simulink model "UAM_GuidanceAndNavigation"  (R2024b)
settings: Solver=VariableStepAuto  StartTime=0.0  StopTime=10.0  RelTol=1e-3
undefined symbols (not defined in the file): Earth, WGS84
libraries: robotcorelib x2, simulink x1, uavalgslib x1, mspfiltlib x1, simulink_extras x1, aerolibtransform2 x1
settings Model: DataDictionary=UAM_data.sldd  Creator=admin  LastModifiedBy=USER

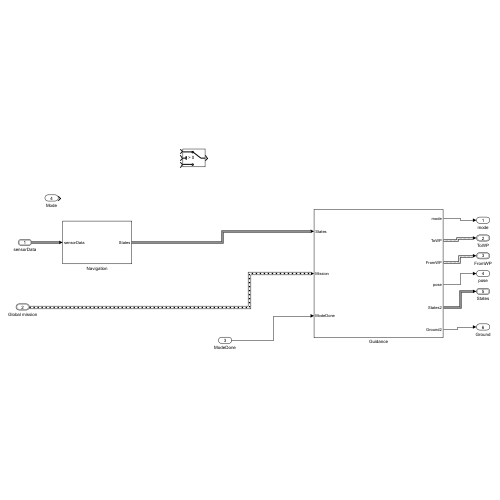
[thumbnail: Simulink's stored preview of the top-level diagram]
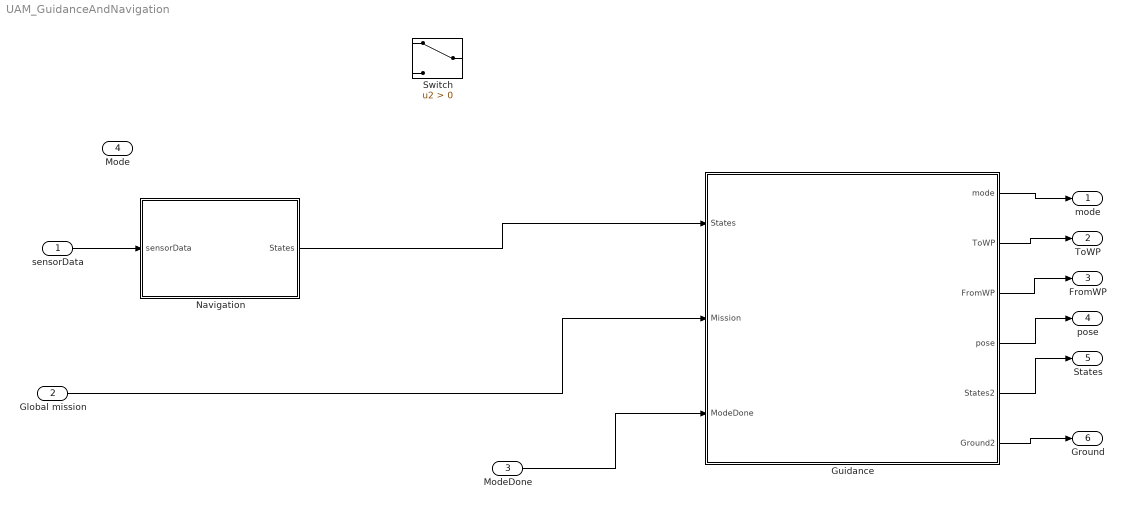
== system UAM_GuidanceAndNavigation ==
  sensorData : Inport  OutDataTypeStr=Bus: sensorData
  Global mission : Inport  Port=2  OutDataTypeStr=Bus: UAVPathManagerBus  PortDimensions=9  BusOutputAsStruct=on
  ModeDone : Inport  Port=3  OutDataTypeStr=uint8
  Mode : Inport  Port=4  OutDataTypeStr=Enum: FlightModeType
  Guidance : Subsystem
  Navigation : Subsystem
  Switch : Switch  Criteria=u2 > Threshold  SaturateOnIntegerOverflow=off  InputSameDT=off
  mode : Outport  BusOutputAsStruct=on
  ToWP : Outport  Port=2  OutDataTypeStr=Bus: UAVPathManagerBus
  FromWP : Outport  Port=3  OutDataTypeStr=Bus: UAVPathManagerBus
  pose : Outport  Port=4
  States : Outport  Port=5  OutDataTypeStr=Bus: GuidanceStates
  Ground : Outport  Port=6
  wires:
  Global mission/1 -> Guidance/2(Mission)
  Navigation/1(States) -> Guidance/1(States)
  sensorData/1 -> Navigation/1(sensorData)
  Guidance/1(mode) -> mode/1
  Guidance/2(ToWP) -> ToWP/1
  Guidance/3(FromWP) -> FromWP/1
  Guidance/4(pose) -> pose/1
  Guidance/5(States2) -> States/1
  Guidance/6(Ground2) -> Ground/1
  ModeDone/1 -> Guidance/3(ModeDone)

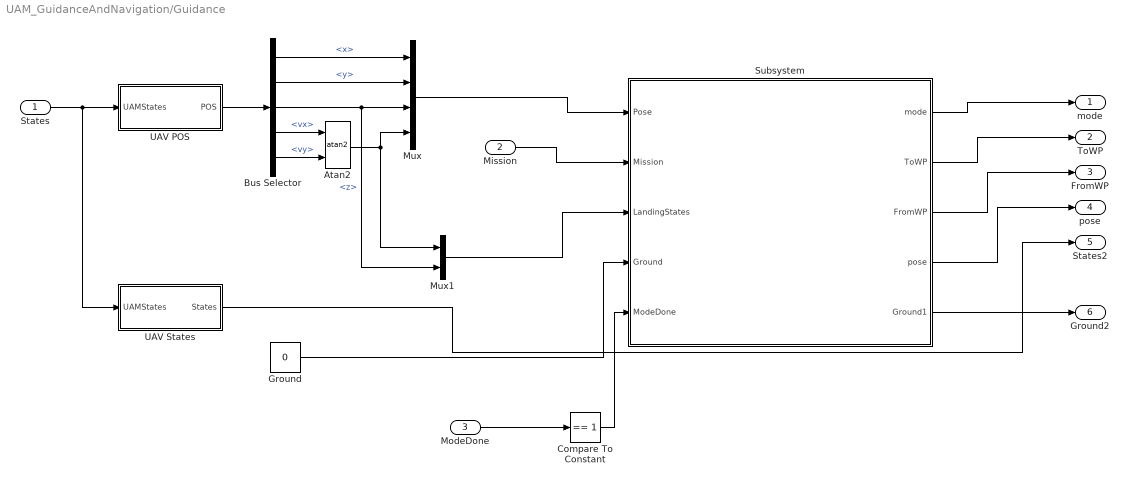
== system UAM_GuidanceAndNavigation/Guidance ==
  States : Inport  OutDataTypeStr=Bus: StateBus
  Mission : Inport  Port=2  OutDataTypeStr=Bus: UAVPathManagerBus
  ModeDone : Inport  Port=3
  Atan2 : Trigonometry  Operator=atan2
  Bus Selector : BusSelector  OutputSignals=x,y,z,vx,vy
  Compare To Constant : simulink/Logic and Bit Operations/Compare To Constant  relop===  const=1  OutDataTypeStr=boolean
  Ground : Constant  Value=0
  Mux : Mux
  Mux1 : Mux  Inputs=2
  Subsystem : Subsystem
  UAV POS : Subsystem
  UAV States : Subsystem
  mode : Outport
  ToWP : Outport  Port=2
  FromWP : Outport  Port=3
  pose : Outport  Port=4
  States2 : Outport  Port=5  OutDataTypeStr=Bus: GuidanceStates
  Ground2 : Outport  Port=6
  wires:
  UAV POS/1(POS) -> Bus Selector/1
  States/1 -> UAV States/1(UAMStates), UAV POS/1(UAMStates)
  Bus Selector/5 -> Atan2/2  "<vy>"
  Bus Selector/4 -> Atan2/1  "<vx>"
  Bus Selector/1 -> Mux/1  "<x>"
  Bus Selector/2 -> Mux/2  "<y>"
  Bus Selector/3 -> Mux1/2, Mux/3  "<z>"
  Atan2/1 -> Mux1/1, Mux/4
  Ground/1 -> Subsystem/4(Ground)
  Mux/1 -> Subsystem/1(Pose)
  Mux1/1 -> Subsystem/3(LandingStates)
  Mission/1 -> Subsystem/2(Mission)
  Subsystem/1(mode) -> mode/1
  Subsystem/5(Ground1) -> Ground2/1
  UAV States/1(States) -> States2/1
  Subsystem/4(pose) -> pose/1
  Subsystem/3(FromWP) -> FromWP/1
  Subsystem/2(ToWP) -> ToWP/1
  ModeDone/1 -> Compare To Constant/1
  Compare To Constant/1 -> Subsystem/5(ModeDone)

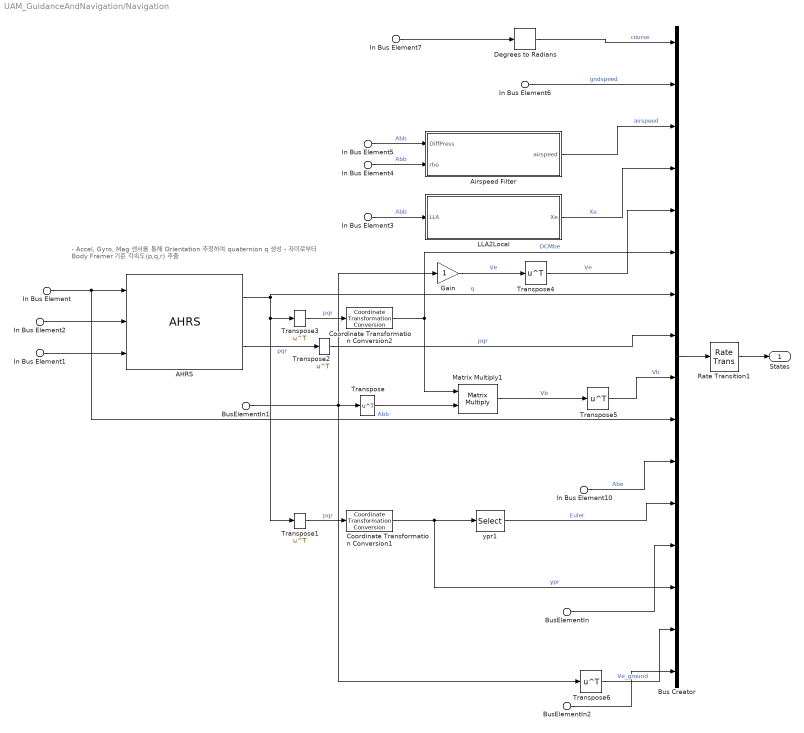
== system UAM_GuidanceAndNavigation/Navigation ==
  note: - Accel, Gyro, Mag 센서를 통해 Orientation 추정하여 quaternion q 생성
      | - 자이로부터 Body Framer 기준 각속도(p,q,r) 추출
  In Bus Element3 : Inport  PortName=sensorData  Element=LLA
  In Bus Element : Inport  PortName=sensorData  Element=Abb
  In Bus Element2 : Inport  PortName=sensorData  Element=Gyro
  In Bus Element1 : Inport  PortName=sensorData  Element=Mag
  BusElementIn1 : Inport  PortName=sensorData  Element=GPSVelocity
  In Bus Element10 : Inport  PortName=sensorData  Element=Abe
  BusElementIn : Inport  PortName=sensorData  Element=RotorParameter
  In Bus Element7 : Inport  PortName=sensorData  Element=GPSCourse
  In Bus Element6 : Inport  PortName=sensorData  Element=gndspeed
  In Bus Element5 : Inport  PortName=sensorData  Element=DiffPress
  In Bus Element4 : Inport  PortName=sensorData  Element=rho
  BusElementIn2 : Inport  PortName=sensorData  Element=RC
  AHRS : mspfiltlib/AHRS  DispRefFrame=NED  DecimationFactor=1  InitialProcessNoise=ahrsfilter.defaultProcessNoise  OrientationFormat=quaternion  SimulateUsing=Interpreted execution  AccelerometerNoise=0.0001924722  GyroscopeNoise=9.1385e-5  MagnetometerNoise=0.1  GyroscopeDriftNoise=3.0462e-13  LinearAccelerationNoise=0.0096236100000000012  MagneticDisturbanceNoise=0.5  LinearAccelerationDecayFactor=0.5  MagneticDisturbanceDecayFactor=0.5  ExpectedMagneticFieldStrength=50
  Airspeed Filter : Subsystem
  Bus Creator : BusCreator  Inputs=16  OutDataTypeStr=Bus: StateBus
  Coordinate Transformation Conversion1 : robotcorelib/Coordinate Transformation Conversion  InputRepresentation=Quaternion  InputEulerSequence=ZYX  ShowTrVecInputPort=on  OutputRepresentation=Euler Angles  OutputEulerSequence=ZYX  ShowTrVecOutputPort=on  SimulateUsing=Interpreted execution
  Coordinate Transformation Conversion2 : robotcorelib/Coordinate Transformation Conversion  InputRepresentation=Quaternion  InputEulerSequence=ZYX  ShowTrVecInputPort=on  OutputRepresentation=Rotation Matrix  OutputEulerSequence=ZYX  ShowTrVecOutputPort=on  SimulateUsing=Interpreted execution
  Degrees to Radians : simulink_extras/Transformations/Degrees to Radians
  Gain : Gain
  LLA2Local : Subsystem
  Matrix Multiply1 : Product  Multiplication=Matrix(*)
  Rate Transition1 : RateTransition
  Transpose{,1..6} (7 alike) : Math  Operator=transpose
  ypr1 : Selector  InputPortWidth=3  IndexOptions=Index vector (dialog)  Indices=[3 2 1]  OutputSizes=1
  States : Outport  OutDataTypeStr=Bus: StateBus
  wires:
  Transpose6/1 -> Bus Creator/15  "Ve_ground"
  In Bus Element/1 -> Bus Creator/10, AHRS/1  "Abb"
  In Bus Element2/1 -> AHRS/2
  ypr1/1 -> Bus Creator/12  "Euler"
  Gain/1 -> Transpose4/1  "Ve"
  Transpose/1 -> Matrix Multiply1/2
  LLA2Local/1(Xe) -> Bus Creator/4  "Xe"
  Matrix Multiply1/1 -> Transpose5/1  "Vb"
  Airspeed Filter/1(airspeed) -> Bus Creator/3  "airspeed"
  BusElementIn1/1 -> Transpose6/1, Transpose/1, Gain/1
  In Bus Element7/1 -> Degrees to Radians/1
  Rate Transition1/1 -> States/1
  In Bus Element6/1 -> Bus Creator/2  "gndspeed"
  Coordinate Transformation Conversion2/1 -> Bus Creator/6, Matrix Multiply1/1  "DCMbe"
  Transpose5/1 -> Bus Creator/9  "Vb"
  Transpose1/1 -> Coordinate Transformation Conversion1/1  "pqr"
  Transpose2/1 -> Bus Creator/8  "pqr"
  Coordinate Transformation Conversion1/1 -> Bus Creator/14, ypr1/1  "ypr"
  AHRS/1 -> Bus Creator/7, Transpose1/1, Transpose3/1  "q"
  In Bus Element10/1 -> Bus Creator/11  "Abe"
  Bus Creator/1 -> Rate Transition1/1
  In Bus Element1/1 -> AHRS/3
  Transpose3/1 -> Coordinate Transformation Conversion2/1  "pqr"
  Degrees to Radians/1 -> Bus Creator/1  "course"
  AHRS/2 -> Transpose2/1  "pqr"
  Transpose4/1 -> Bus Creator/5  "Ve"
  In Bus Element3/1 -> LLA2Local/1(LLA)  "Abb"
  In Bus Element4/1 -> Airspeed Filter/2(rho)  "Abb"
  In Bus Element5/1 -> Airspeed Filter/1(DiffPress)  "Abb"
  BusElementIn/1 -> Bus Creator/13
  BusElementIn2/1 -> Bus Creator/16

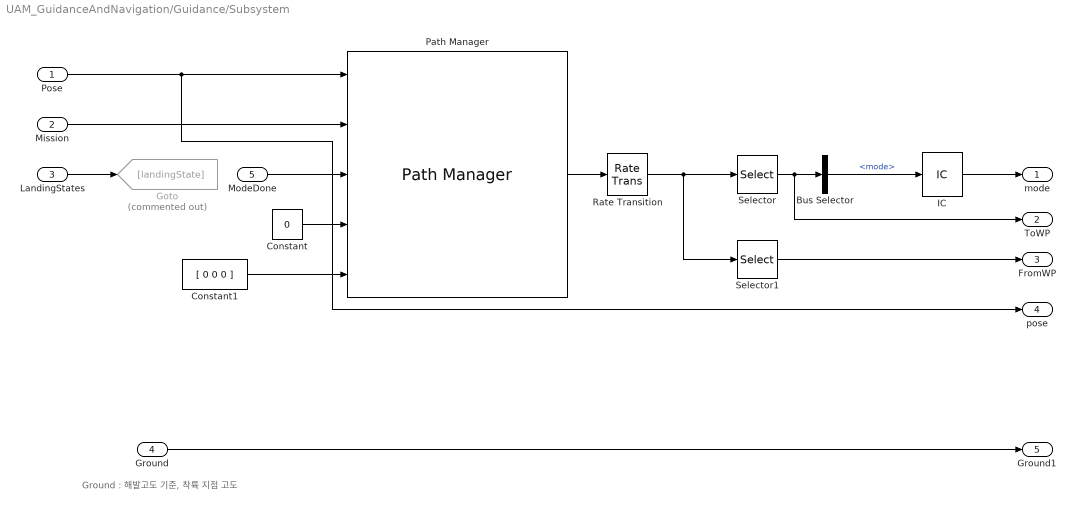
== system UAM_GuidanceAndNavigation/Guidance/Subsystem ==
  note: Ground : 해발고도 기준, 착륙 지점 고도
  Pose : Inport
  Mission : Inport  Port=2  OutDataTypeStr=Bus: UAVPathManagerBus
  LandingStates : Inport  Port=3
  Ground : Inport  Port=4
  ModeDone : Inport  Port=5
  Bus Selector : BusSelector  OutputSignals=mode
  Constant : Constant  Value=0
  Constant1 : Constant  Value=[ 0 0 0 ]  OutDataTypeStr=double
  Goto : Goto  Commented=on  GotoTag=landingState
  IC : InitialCondition
  Path Manager : uavalgslib/Path Manager  UAVType=multirotor  LoiterRadius=25  dataType=double  inputBusName='UAVPathManagerBus'  SimulateUsing=Interpreted execution
  Rate Transition : RateTransition
  Selector : Selector  InputPortWidth=2  IndexOptions=Index vector (dialog)  Indices=1  OutputSizes=1
  Selector1 : Selector  InputPortWidth=2  IndexOptions=Index vector (dialog)  Indices=2  OutputSizes=1
  mode : Outport
  ToWP : Outport  Port=2
  FromWP : Outport  Port=3
  pose : Outport  Port=4
  Ground1 : Outport  Port=5
  wires:
  Pose/1 -> pose/1, Path Manager/1
  LandingStates/1 -> Goto/1
  Constant/1 -> Path Manager/4
  Mission/1 -> Path Manager/2
  Path Manager/1 -> Rate Transition/1
  Rate Transition/1 -> Selector1/1, Selector/1
  Constant1/1 -> Path Manager/5
  Selector/1 -> ToWP/1, Bus Selector/1
  Ground/1 -> Ground1/1
  Bus Selector/1 -> IC/1  "<mode>"
  IC/1 -> mode/1
  Selector1/1 -> FromWP/1
  ModeDone/1 -> Path Manager/3

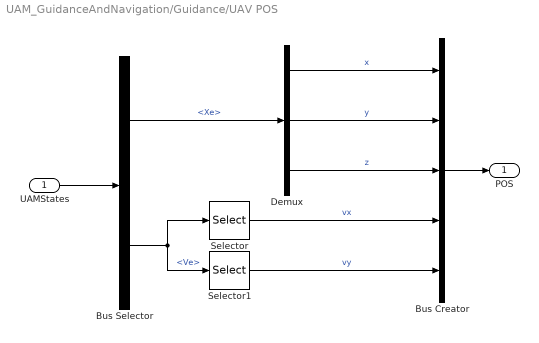
== system UAM_GuidanceAndNavigation/Guidance/UAV POS ==
  UAMStates : Inport  OutDataTypeStr=Bus: StateBus
  Bus Creator : BusCreator  Inputs=5
  Bus Selector : BusSelector  OutputSignals=Xe,Ve
  Demux : Demux  Outputs=3
  Selector : Selector  InputPortWidth=3  IndexOptions=Index vector (dialog)  Indices=[1]  OutputSizes=1
  Selector1 : Selector  InputPortWidth=3  IndexOptions=Index vector (dialog)  Indices=[2]  OutputSizes=1
  POS : Outport
  wires:
  UAMStates/1 -> Bus Selector/1
  Bus Selector/1 -> Demux/1  "<Xe>"
  Demux/1 -> Bus Creator/1  "x"
  Demux/2 -> Bus Creator/2  "y"
  Demux/3 -> Bus Creator/3  "z"
  Bus Selector/2 -> Selector/1, Selector1/1  "<Ve>"
  Selector/1 -> Bus Creator/4  "vx"
  Selector1/1 -> Bus Creator/5  "vy"
  Bus Creator/1 -> POS/1

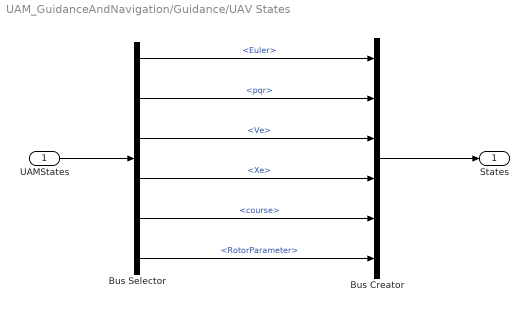
== system UAM_GuidanceAndNavigation/Guidance/UAV States ==
  UAMStates : Inport
  Bus Creator : BusCreator  Inputs=6
  Bus Selector : BusSelector  OutputSignals=Euler,pqr,Ve,Xe,course,RotorParameter
  States : Outport
  wires:
  UAMStates/1 -> Bus Selector/1
  Bus Selector/3 -> Bus Creator/3  "<Ve>"
  Bus Selector/1 -> Bus Creator/1  "<Euler>"
  Bus Selector/2 -> Bus Creator/2  "<pqr>"
  Bus Selector/4 -> Bus Creator/4  "<Xe>"
  Bus Selector/5 -> Bus Creator/5  "<course>"
  Bus Creator/1 -> States/1
  Bus Selector/6 -> Bus Creator/6  "<RotorParameter>"

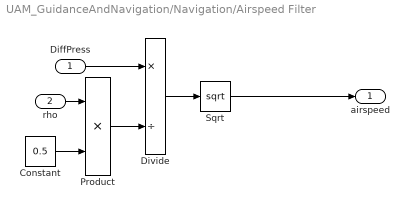
== system UAM_GuidanceAndNavigation/Navigation/Airspeed Filter ==
  DiffPress : Inport
  rho : Inport  Port=2
  Constant : Constant  Value=0.5
  Divide : Product  Inputs=*/
  Product : Product
  Sqrt : Sqrt
  airspeed : Outport
  wires:
  Sqrt/1 -> airspeed/1
  Divide/1 -> Sqrt/1
  DiffPress/1 -> Divide/1
  Product/1 -> Divide/2
  rho/1 -> Product/1
  Constant/1 -> Product/2

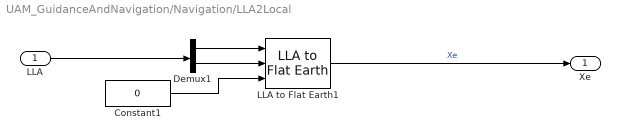
== system UAM_GuidanceAndNavigation/Navigation/LLA2Local ==
  LLA : Inport
  Constant1 : Constant  Value=0
  Demux1 : Demux  Outputs=[2 1]
  LLA to Flat Earth1 : aerolibtransform2/LLA to Flat Earth  units=Metric (MKS)  ptype=Earth (WGS84)  F=1/298.257223563  R=6378137  refPosPort=off  LL0=[0 0]  psi=0
  Xe : Outport
  wires:
  LLA/1 -> Demux1/1
  LLA to Flat Earth1/1 -> Xe/1  "Xe"
  Demux1/2 -> LLA to Flat Earth1/2
  Demux1/1 -> LLA to Flat Earth1/1
  Constant1/1 -> LLA to Flat Earth1/3
